simulink model "model2"  (R2017a)
settings: Solver=VariableStepAuto  StartTime=0.0  StopTime=80  RelTol=1e-3
values from neighbouring files (symbols this model uses):
  motor = gm9434    [motor_code.m]
undefined symbols (not defined in the file or in its folder): current_ctrl, vest
libraries: simulink x4
settings Model: Creator=rodrigo  LastModifiedBy=rodrigo

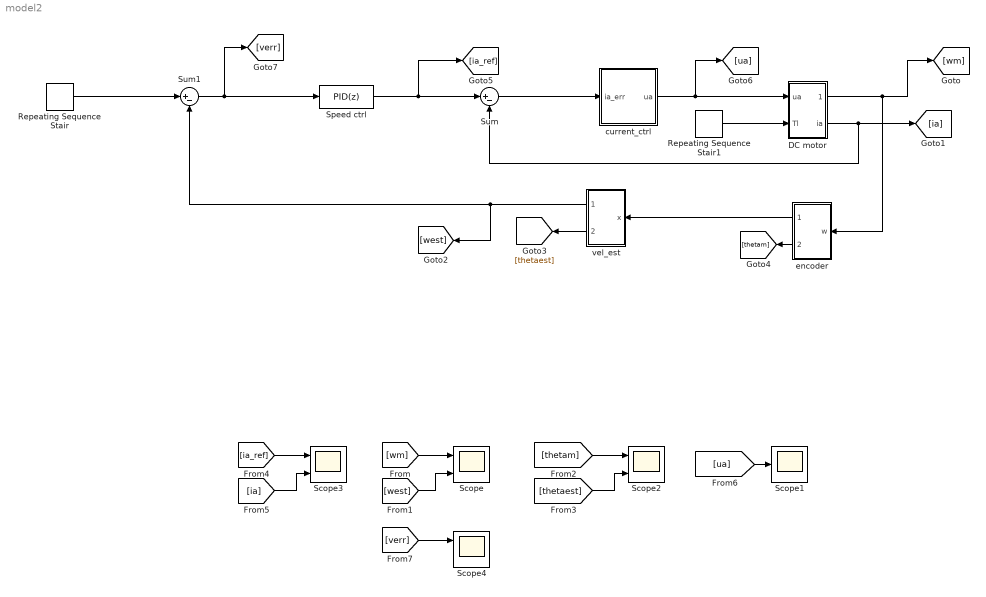
== system model2 ==
  DC motor : Subsystem
  Repeating Sequence Stair : simulink/Sources/Repeating Sequence Stair  OutValues=[50 80 50 0 -20 0 10].'  tsamp=4  OutMin=[]  OutMax=[]  OutDataTypeStr=double  OutputDataTypeScalingMode=double  OutDataType=fixdt(0,8)  ConRadixGroup=Best Precision: Vector-wise  OutScaling=2^-12
  Repeating Sequence Stair1 : simulink/Sources/Repeating Sequence Stair  OutValues=1e-5*[50 80 50 0 -20 0 10].'  tsamp=4  OutMin=[]  OutMax=[]  OutDataTypeStr=double  OutputDataTypeScalingMode=double  OutDataType=fixdt(0,8)  ConRadixGroup=Best Precision: Vector-wise  OutScaling=2^-12
  Scope{,2..4} (4 alike) : Scope  NumInputPorts=2
  Scope1 : Scope
  Speed ctrl : simulink/Continuous/PID Controller  Controller=PID  TimeDomain=Discrete-time  SampleTime=current_ctrl.Ts*30  IntegratorMethod=Forward Euler  FilterMethod=Forward Euler  Form=Parallel  UseFilter=off  ControllerParametersSource=internal  P=0.0008  I=0.002  D=0  N=100  InitialConditionSource=internal  InitialConditionForIntegrator=0  InitialConditionForFilter=0  ExternalReset=none  ZeroCross=off  LimitOutput=off  UpperSaturationLimit=12  LowerSaturationLimit=-12  LinearizeAsGain=off  AntiWindupMode=back-calculation  Kb=1  TrackingMode=off  Kt=1  PParamMin=[]  PParamMax=[]  IParamMin=[]  IParamMax=[]  DParamMin=[]  DParamMax=[]  NParamMin=[]  NParamMax=[]  KbParamMin=[]  KbParamMax=[]  KtParamMin=[]  KtParamMax=[]  POutMin=[]  POutMax=[]  IOutMin=[]  IOutMax=[]  DOutMin=[]  DOutMax=[]  NOutMin=[]  NOutMax=[]  KbOutMin=[]  KbOutMax=[]  KtOutMin=[]  KtOutMax=[]  IntegratorOutMin=[]  IntegratorOutMax=[]  FilterOutMin=[]  FilterOutMax=[]  SumOutMin=[]  SumOutMax=[]  SumI1OutMin=[]  SumI1OutMax=[]  SumI2OutMin=[]  SumI2OutMax=[]  SumI3OutMin=[]  SumI3OutMax=[]  SumDOutMin=[]  SumDOutMax=[]  SaturationOutMin=[]  SaturationOutMax=[]  IntegratorContinuousStateAttributes=''  IntegratorStateMustResolveToSignalObject=off  IntegratorRTWStateStorageClass=Auto  FilterContinuousStateAttributes=''  FilterStateMustResolveToSignalObject=off  FilterRTWStateStorageClass=Auto  DifferentiatorICPrevScaledInput=0  DifferentiatorOutMin=[]  DifferentiatorOutMax=[]  InitialConditionSetting=State (most efficient)
  Sum : Sum  Inputs=|+-
  Sum1 : Sum  Inputs=|+-
  current_ctrl : Subsystem
  encoder : Subsystem
  vel_est : Subsystem
  wires:
  current_ctrl/1(ua) -> [ua], DC motor/1(ua)
  DC motor/2(ia) -> [ia], Sum/2
  Sum/1 -> current_ctrl/1(ia_err)
  DC motor/1(wm) -> encoder/1(w), [wm]
  [thetam] -> Scope2/1
  [thetaest] -> Scope2/2
  [ia] -> Scope3/2
  vel_est/2(xest) -> [thetaest]
  [ia_ref] -> Scope3/1
  [wm] -> Scope/1
  encoder/2(theta) -> [thetam]
  vel_est/1(vest) -> [west], Sum1/2
  [ua] -> Scope1/1
  Sum1/1 -> [verr], Speed ctrl/1
  [verr] -> Scope4/1
  encoder/1(theta_q) -> vel_est/1(x)
  Speed ctrl/1 -> [ia_ref], Sum/1
  [west] -> Scope/2
  Repeating Sequence Stair1/1 -> DC motor/2(Tl)
  Repeating Sequence Stair/1 -> Sum1/1

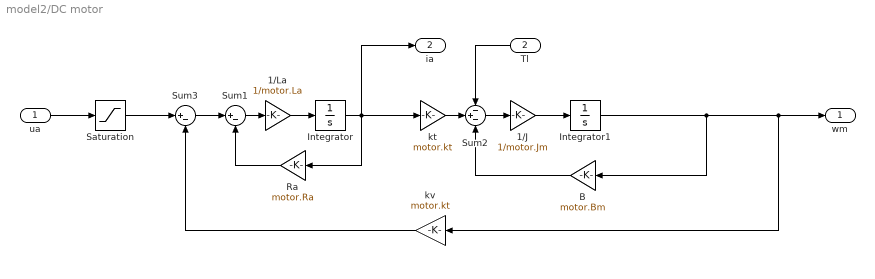
== system model2/DC motor ==
  ua : Inport
  Tl : Inport  Port=2
  1/J : Gain  Gain=1/motor.Jm
  1/La : Gain  Gain=1/motor.La
  B : Gain  Gain=motor.Bm
  Integrator : Integrator  ZeroCross=off
  Integrator1 : Integrator
  Ra : Gain  Gain=motor.Ra
  Saturation : Saturate  UpperLimit=12  LowerLimit=-12
  Sum1 : Sum  Inputs=|+-
  Sum2 : Sum  Inputs=-+-
  Sum3 : Sum  Inputs=|+-
  kt : Gain  Gain=motor.kt
  kv : Gain  Gain=motor.kt
  wm : Outport
  ia : Outport  Port=2
  wires:
  1/J/1 -> Integrator1/1
  Sum2/1 -> 1/J/1
  Integrator1/1 -> B/1, wm/1, kv/1
  ua/1 -> Saturation/1
  Integrator/1 -> kt/1, Ra/1, ia/1
  Ra/1 -> Sum1/2
  1/La/1 -> Integrator/1
  Tl/1 -> Sum2/1
  kv/1 -> Sum3/2
  Sum3/1 -> Sum1/1
  kt/1 -> Sum2/2
  Sum1/1 -> 1/La/1
  Saturation/1 -> Sum3/1
  B/1 -> Sum2/3

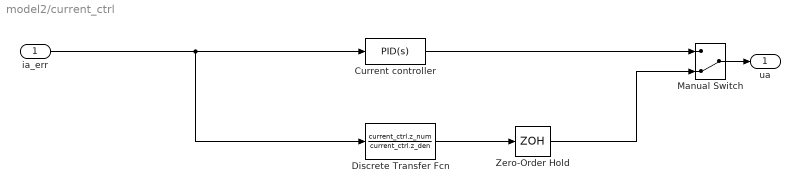
== system model2/current_ctrl ==
  ia_err : Inport
  Current controller : simulink/Continuous/PID Controller  Controller=PID  TimeDomain=Continuous-time  SampleTime=-1  IntegratorMethod=Forward Euler  FilterMethod=Forward Euler  Form=Parallel  UseFilter=off  ControllerParametersSource=internal  P=current_ctrl.kp  I=current_ctrl.ki  D=0  N=100  InitialConditionSource=internal  InitialConditionForIntegrator=0  InitialConditionForFilter=0  ExternalReset=none  ZeroCross=off  LimitOutput=off  UpperSaturationLimit=12  LowerSaturationLimit=-12  LinearizeAsGain=off  AntiWindupMode=back-calculation  Kb=1  TrackingMode=off  Kt=1  PParamMin=[]  PParamMax=[]  IParamMin=[]  IParamMax=[]  DParamMin=[]  DParamMax=[]  NParamMin=[]  NParamMax=[]  KbParamMin=[]  KbParamMax=[]  KtParamMin=[]  KtParamMax=[]  POutMin=[]  POutMax=[]  IOutMin=[]  IOutMax=[]  DOutMin=[]  DOutMax=[]  NOutMin=[]  NOutMax=[]  KbOutMin=[]  KbOutMax=[]  KtOutMin=[]  KtOutMax=[]  IntegratorOutMin=[]  IntegratorOutMax=[]  FilterOutMin=[]  FilterOutMax=[]  SumOutMin=[]  SumOutMax=[]  SumI1OutMin=[]  SumI1OutMax=[]  SumI2OutMin=[]  SumI2OutMax=[]  SumI3OutMin=[]  SumI3OutMax=[]  SumDOutMin=[]  SumDOutMax=[]  SaturationOutMin=[]  SaturationOutMax=[]  IntegratorContinuousStateAttributes=''  IntegratorStateMustResolveToSignalObject=off  IntegratorRTWStateStorageClass=Auto  FilterContinuousStateAttributes=''  FilterStateMustResolveToSignalObject=off  FilterRTWStateStorageClass=Auto  DifferentiatorICPrevScaledInput=0  DifferentiatorOutMin=[]  DifferentiatorOutMax=[]  InitialConditionSetting=State (most efficient)
  Discrete Transfer Fcn : DiscreteTransferFcn  Numerator=current_ctrl.z_num  Denominator=current_ctrl.z_den  SampleTime=current_ctrl.Ts
  Manual Switch : ManualSwitch  CurrentSetting=0
  Zero-Order Hold : ZeroOrderHold  SampleTime=current_ctrl.Ts
  ua : Outport
  wires:
  ia_err/1 -> Discrete Transfer Fcn/1, Current controller/1
  Current controller/1 -> Manual Switch/1
  Discrete Transfer Fcn/1 -> Zero-Order Hold/1
  Zero-Order Hold/1 -> Manual Switch/2
  Manual Switch/1 -> ua/1

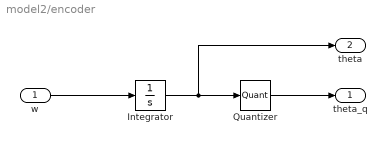
== system model2/encoder ==
  w : Inport
  Integrator : Integrator
  Quantizer : Quantizer  QuantizationInterval=encoder
  theta_q : Outport
  theta : Outport  Port=2
  wires:
  Quantizer/1 -> theta_q/1
  w/1 -> Integrator/1
  Integrator/1 -> theta/1, Quantizer/1

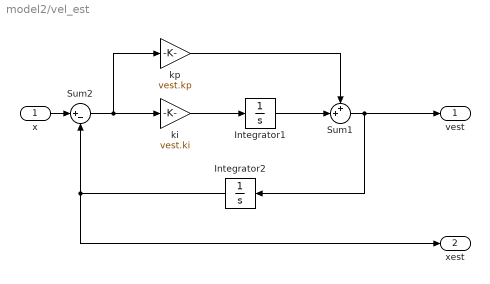
== system model2/vel_est ==
  x : Inport
  Integrator1 : Integrator  ZeroCross=off
  Integrator2 : Integrator
  Sum1 : Sum  Inputs=++|
  Sum2 : Sum  Inputs=|+-
  ki : Gain  Gain=vest.ki
  kp : Gain  Gain=vest.kp
  vest : Outport
  xest : Outport  Port=2
  wires:
  ki/1 -> Integrator1/1
  Sum2/1 -> kp/1, ki/1
  Integrator2/1 -> xest/1, Sum2/2
  kp/1 -> Sum1/1
  Integrator1/1 -> Sum1/2
  x/1 -> Sum2/1
  Sum1/1 -> vest/1, Integrator2/1
